simulink model "stateflow_3_stm_car"  (R2021b)
settings: Solver=VariableStepAuto  StartTime=0.0  StopTime=inf  RelTol=1e-3
values from neighbouring files (symbols this model uses):
  DD = 3.0    [stm_car.sldd]
  NN = 2.0    [stm_car.sldd]
  PP = 0.0    [stm_car.sldd]
  RR = 1.0    [stm_car.sldd]
settings Model: DataDictionary=stm_car.sldd  Creator=fredric  LastModifiedBy=fredric

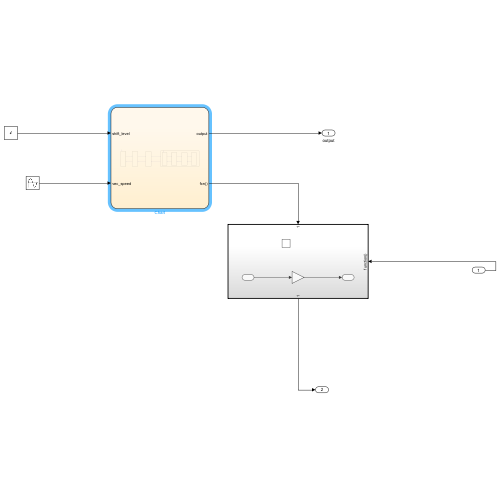
[thumbnail: Simulink's stored preview of the top-level diagram]
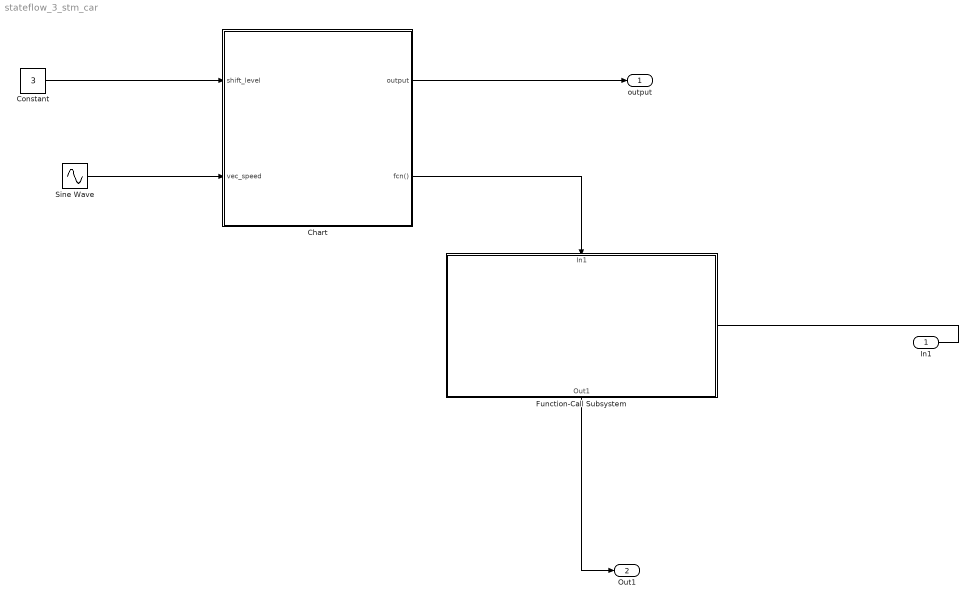
== system stateflow_3_stm_car ==
  In1 : Inport
  Chart : Stateflow chart  TreatAsAtomicUnit=on
  Constant : Constant  Value=3
  Function-Call Subsystem : Subsystem  TreatAsAtomicUnit=on
  Sine Wave : Sin  Amplitude=80  SampleTime=0
  output : Outport
  Out1 : Outport  Port=2
  wires:
  Sine Wave/1 -> Chart/2(vec_speed)
  Constant/1 -> Chart/1(shift_level)
  Chart/2(fcn()) -> Function-Call Subsystem/1(In1)
  In1/1 -> Function-Call Subsystem/Trigger
  Chart/1(output) -> output/1
  Function-Call Subsystem/1(Out1) -> Out1/1

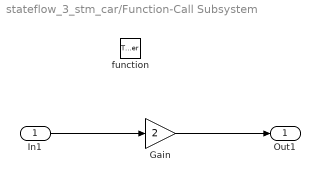
== system stateflow_3_stm_car/Function-Call Subsystem ==
  In1 : Inport
  function : TriggerPort  TriggerType=function-call  VariantControl=(inherit)
  Gain : Gain  Gain=2
  Out1 : Outport
  wires:
  In1/1 -> Gain/1
  Gain/1 -> Out1/1

== stateflow chart stateflow_3_stm_car/Chart ==
  state D
    state D1
      en:
      output=10;
    state D2
      en:
      output=20;
    state D3
      en:
      output=30;
    state D4
      en:
      output=40;
    (default) -> D1
    D1 -> D2 : [vec_speed>30]
    D2 -> D3 [order 1] : [vec_speed>50]
    D3 -> D4 [order 1] : [vec_speed>70]
    D2 -> D1 [order 2] : [vec_speed<25]
    D3 -> D2 [order 2] : [vec_speed<45]
    D4 -> D3 : [vec_speed<65]
  state P
  state R
    en:
    fcn;
    du:
    fcn;
  state N
  (default) -> P
  P -> R : [ shift_level==RR ]
  N -> D [order 1] : [ shift_level==DD ]
  R -> N [order 1] : [ shift_level==NN ]
  D -> N : [ shift_level==NN ]
  N -> R [order 2] : [ shift_level==RR ]
  R -> P [order 2] : [ shift_level==PP ]
  data: shift_level input; vec_speed input; output output; PP parameter; RR parameter; NN parameter; DD parameter
  events: fcn output FUNCTION_CALL_EVENT
